simulink model "F16_LongDyn_pub"  (Simulink 7.3)
settings: Solver=ode45  StartTime=0.0  StopTime=Tsim  MaxStep=1e-3  RelTol=1e-5
InitFcn:
  | aoa_cas_init
values from neighbouring files (symbols this model uses):
  A = [-1.9311e-2   8.8157e+0 -3.2170e+1 -5.7499e-1 ... (first row only)    [aoa_cas_init.m]
  B = [ 1.7370e-1 ... (first row only)    [aoa_cas_init.m]
  C = [0.000000e+0       180/pi  0.000000e+0  0.000000e+0 ... (first row only)    [aoa_cas_init.m]
  D = zeros(2,1)    [aoa_cas_init.m]
  k_alpha = -0.08    [aoa_cas_init.m]
  k_q = -0.5    [aoa_cas_init.m]
  ki = -1.5    [aoa_cas_init.m]
  kp = -1.5    [aoa_cas_init.m]
  tau_a = 1/20.2    (= 0.049504950495)    [aoa_cas_init.m]
  tau_f = 0.1    [aoa_cas_init.m]
settings Model: Creator=vldobr  LastModifiedBy=vldobr

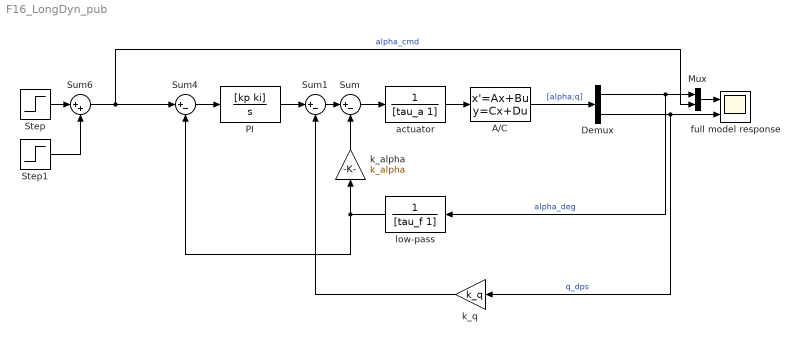
== system F16_LongDyn_pub ==
  A/C : StateSpace  A=A  B=B  C=C  D=D
  Demux : Demux  Outputs=2
  Mux : Mux  Inputs=2
  PI : TransferFcn  Numerator=[kp ki]  Denominator=[1 0]
  Step : Step  SampleTime=0
  Step1 : Step  Time=9  After=-1  SampleTime=0
  Sum : Sum  Inputs=|+-
  Sum1 : Sum  Inputs=|+-
  Sum4 : Sum  Inputs=|+-
  Sum6 : Sum  Inputs=|++
  actuator : TransferFcn  Denominator=[tau_a 1]
  full model response : Scope  NumInputPorts=2
      settings: YMin=-5~-5  YMax=5~5  SaveName=NLData
  k_alpha : Gain  Gain=k_alpha
  k_q : Gain  Gain=k_q
  "low-pass " : TransferFcn  Denominator=[tau_f 1]
  wires:
  A/C/1 -> Demux/1  "[alpha;q]"
  actuator/1 -> A/C/1
  Demux/1 -> "low-pass "/1, Mux/1  "alpha_deg"
  Demux/2 -> full model response/2, k_q/1  "q_dps"
  "low-pass "/1 -> k_alpha/1, Sum4/2
  Sum/1 -> actuator/1
  k_alpha/1 -> Sum/2
  Sum1/1 -> Sum/1
  k_q/1 -> Sum1/2
  PI/1 -> Sum1/1
  Sum4/1 -> PI/1
  Step/1 -> Sum6/1
  Mux/1 -> full model response/1
  Sum6/1 -> Sum4/1, Mux/2  "alpha_cmd"
  Step1/1 -> Sum6/2
